simulink model "cheapsensor"  (R2022b)
settings: Solver=VariableStepAuto  StartTime=0.0  StopTime=20  RelTol=1e-3
values from neighbouring files (symbols this model uses):
  A = parameters{1}    [cheap.m]
  B = parameters{2}    [cheap.m]
  C = parameters{3}    [cheap.m]
  K1 = K_calculated(:,1:6)    [cheap.m]
  K2 = K_calculated(:,7:9)    [cheap.m]
  L = real(L)    [cheap.m]
  w = [-1;1]    [cheap.m]
  x0 = parameters{5}    [cheap.m]
  ysp = parameters{7}    [cheap.m]
settings Model: Creator=wyton  LastModifiedBy=wanrylin
settings SolverCC: AlgebraicLoopSolver=TrustRegion
settings DebuggingCC: UnconnectedInputMsg=warning  UnconnectedOutputMsg=warning  UnconnectedLineMsg=warning  SFMachineParentedDataDiag=warning
settings ModelReferenceCC: EnableRefExpFcnMdlSchedulingChecks=on
settings RTWCC: DLArmComputeVersion=19.05

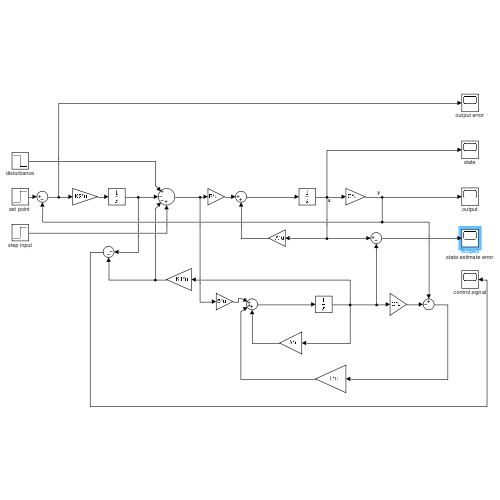
[thumbnail: Simulink's stored preview of the top-level diagram]
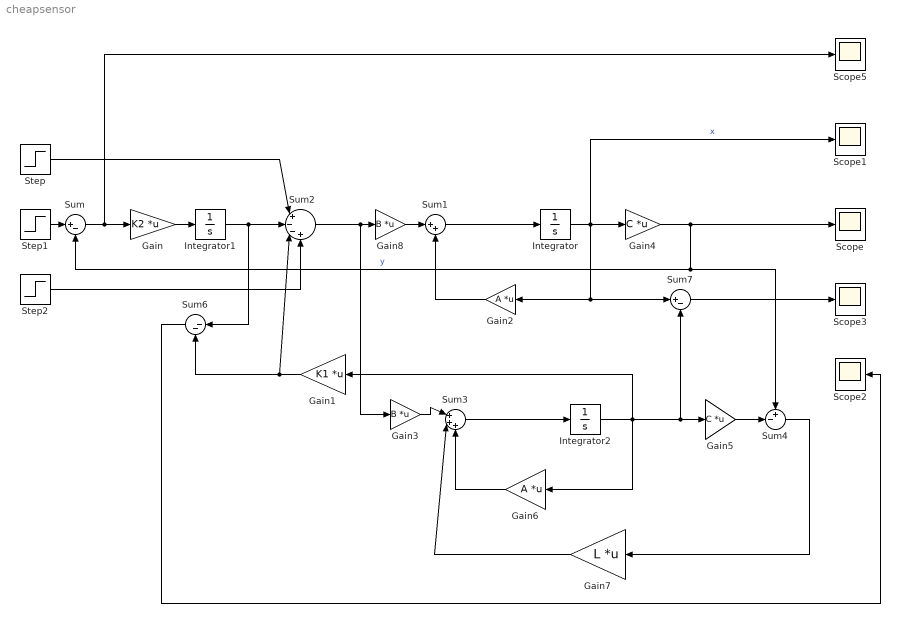
== system cheapsensor ==
  Gain : Gain  Gain=K2  Multiplication=Matrix(K*u)
  Gain1 : Gain  Gain=K1  Multiplication=Matrix(K*u)
  Gain2 : Gain  Gain=A  Multiplication=Matrix(K*u)
  Gain3 : Gain  Gain=B  Multiplication=Matrix(K*u)
  Gain4 : Gain  Gain=C  Multiplication=Matrix(K*u)
  Gain5 : Gain  Gain=C  Multiplication=Matrix(K*u)
  Gain6 : Gain  Gain=A  Multiplication=Matrix(K*u)
  Gain7 : Gain  Gain=L  Multiplication=Matrix(K*u)
  Gain8 : Gain  Gain=B  Multiplication=Matrix(K*u)
  Integrator : Integrator  InitialCondition=x0
  Integrator1 : Integrator
  Integrator2 : Integrator
  Scope{,1..3,5} (5 alike) : Scope
      Scope settings: AttributesFormatString=output
      Scope1 settings: AttributesFormatString=state
      Scope2 settings: AttributesFormatString=control signal
      Scope3 settings: AttributesFormatString=state estimate error
      Scope5 settings: AttributesFormatString=output error
  Step : Step  Time=10  Before=[0;0]  After=w  SampleTime=0
      settings: AttributesFormatString=disturbance
  Step1 : Step  Time=0  Before=[0;0;0]  After=ysp  SampleTime=0
      settings: AttributesFormatString=set point
  Step2 : Step  Time=0  Before=[0,0]  After=[1,0]  SampleTime=0
      settings: AttributesFormatString=step input
  Sum : Sum  Inputs=|+-
  Sum1 : Sum  Inputs=|++
  Sum2 : Sum  Inputs=|+--+
  Sum3 : Sum  Inputs=|+++
  Sum4 : Sum  Inputs=+-|
  Sum6 : Sum  Inputs=|--
  Sum7 : Sum  Inputs=|+-
  wires:
  Sum1/1 -> Integrator/1
  Gain2/1 -> Sum1/2
  Integrator/1 -> Gain2/1, Sum7/1, Scope1/1, Gain4/1  "x"
  Gain4/1 -> Scope/1, Sum/2, Sum4/1  "y"
  Gain3/1 -> Sum3/1
  Sum3/1 -> Integrator2/1
  Integrator2/1 -> Sum7/2, Gain5/1, Gain1/1, Gain6/1
  Gain6/1 -> Sum3/3
  Gain5/1 -> Sum4/2
  Gain7/1 -> Sum3/2
  Sum4/1 -> Gain7/1
  Gain1/1 -> Sum6/2, Sum2/3
  Gain8/1 -> Sum1/1
  Sum2/1 -> Gain8/1, Gain3/1
  Sum/1 -> Gain/1, Scope5/1
  Gain/1 -> Integrator1/1
  Integrator1/1 -> Sum6/1, Sum2/2
  Step/1 -> Sum2/1
  Sum6/1 -> Scope2/1
  Sum7/1 -> Scope3/1
  Step1/1 -> Sum/1
  Step2/1 -> Sum2/4
